simulink model "bldc0"  (R2022b)
settings: Solver=ode1  StartTime=0.0  StopTime=0.2  FixedStep=ctrlConst.TsSwitch  MaxStep=1e-6  RelTol=1e-3  EnableMultiTasking=on
values from neighbouring files (symbols this model uses):
  f32_P_AngleCompCur = 5461.0    [bldc.sldd]
  f32_P_AngleCompVol = 1.5    [bldc.sldd]
  f32_P_CurMax_A = 43.0    [bldc.sldd]
  f32_P_DeadPrd = 80.0    [bldc.sldd]
  f32_P_FwcCurMax_A = 54.2    [bldc.sldd]
  f32_P_fwcKi = 0.3    [bldc.sldd]
  f32_P_fwcKp = 11.0    [bldc.sldd]
  f32_P_IdInIF_A = -5.0    [bldc.sldd]
  f32_P_IdKi = 0.00010825    [bldc.sldd]
  f32_P_IdKp = 0.02    [bldc.sldd]
  f32_P_IdqFilter = 1250.0    [bldc.sldd]
  f32_P_IqKi = 0.00010825    [bldc.sldd]
  f32_P_IqKp = 0.02    [bldc.sldd]
  f32_P_MaxTrq_Nm = 1500.0    [bldc.sldd]
  f32_P_MinTrq_Nm = -1500.0    [bldc.sldd]
  f32_P_Modulation = 0.95    [bldc.sldd]
  f32_P_MotorPhi = 0.0026    [bldc.sldd]
  f32_P_PWMFreq = 10000.0    [bldc.sldd]
  f32_P_SpdNegKi = 10.0    [bldc.sldd]
  f32_P_SpdNegKp = 100.0    [bldc.sldd]
  f32_P_SpdNeglimit_rpm = -6000.0    [bldc.sldd]
  f32_P_SpdPosKi = 10.0    [bldc.sldd]
  f32_P_SpdPosKp = 100.0    [bldc.sldd]
  f32_P_SpdPoslimit_rpm = 6000.0    [bldc.sldd]
  f32_P_SpeedKi = 2.5E-6    [bldc.sldd]
  f32_P_SpeedKp = 0.02    [bldc.sldd]
  f32_P_SpeedPiMax = 1.5    [bldc.sldd]
  f32_P_SpeedPiMin = -1.5    [bldc.sldd]
  f32_P_Uqmax = 0.955    [bldc.sldd]
  u16_P_MotorPair = 4.0    [bldc.sldd]
undefined symbols (not defined in the file or in its folder): ECM
libraries: simulink x6, spsabctodq0Lib x1
(part 1 of 2)
settings Model: Creator=M00039784  LastModifiedBy=M00039784
settings SolverCC: AlgebraicLoopSolver=TrustRegion  InsertRTBMode=Never (minimum delay)
settings DataIOCC: LimitDataPoints=on  SaveFormat=Array  SaveOutput=off  SaveTime=off
settings OptimizationCC: DefaultParameterBehavior=Inlined  UseDivisionForNetSlopeComputation=on  UseFloatMulNetSlope=on  DefaultUnderspecifiedDataType=single  InlineInvariantSignals=on  PassReuseOutputArgsAs=Individual arguments  ExpressionDepthLimit=2147483647  ZeroExternalMemoryAtStartup=off  ZeroInternalMemoryAtStartup=off  NoFixptDivByZeroProtection=on  EfficientFloat2IntCast=on  LifeSpan=1  EfficientTunableParamExpr=on
settings DebuggingCC: ReadBeforeWriteMsg=DisableAll  WriteAfterWriteMsg=DisableAll  WriteAfterReadMsg=DisableAll  AlgebraicLoopMsg=none  MultiTaskDSMMsg=none  SingleTaskRateTransMsg=error  IntegerOverflowMsg=none  ParameterPrecisionLossMsg=none  FcnCallInpInsideContextMsg=warning  BusObjectLabelMismatch=none  AssertControl=DisableAll  AllowSymbolicDim=off  StateNameClashWarn=warning  SFUnexpectedBacktrackingDiag=warning  SFNoUnconditionalDefaultTransitionDiag=warning  SFExecutionAtInitializationDiag=none  SFMachineParentedDataDiag=warning  IntegerSaturationMsg=none  UnitsInconsistencyMsg=none  ArithmeticOperatorsInVariantConditions=warning
settings HardwareCC: ProdBitPerPointer=32  ProdBitPerSizeT=32  ProdBitPerPtrDiffT=32  ProdLargestAtomicFloat=None  ProdWordSize=32  ProdHWDeviceType=Infineon->TriCore
settings ModelReferenceCC: UpdateModelReferenceTargets=IfOutOfDate  EnableRefExpFcnMdlSchedulingChecks=on  ModelReferenceNumInstancesAllowed=Single  PropagateSignalLabelsOutOfModel=off
settings SFSimCC: SFSimEcho=off  SimUseLocalCustomCode=off  SimGenImportedTypeDefs=on  MATLABDynamicMemAlloc=off  CustomCodeUndefinedFunction=UseInterfaceOnly
settings RTWCC: Description=Embedded Coder  SystemTargetFile=ert.tlc  GenCodeOnly=on  GenerateMakefile=off  TemplateMakefile=ec_target.tmf  RTWVerbose=off  RTWUseLocalCustomCode=off  PortableWordSizes=on  CodeExecutionProfiling=on  CodeProfilingSaveOptions=AllData  CodeProfilingInstrumentation=detailed
settings CodeAppCC: ForceParamTrailComments=on  IgnoreCustomStorageClasses=off  IgnoreTestpoints=on  MaxIdLength=64  SimulinkDataObjDesc=on  MATLABFcnDesc=on  CustomSymbolStrGlobalVar=pmsmfoc_rt$N$M  CustomSymbolStrType=pmsmfoc_$N$M  CustomSymbolStrFcn=$N$M$F  CustomSymbolStrFcnArg=$I$N$M  CustomSymbolStrMacro=$N$M  InsertBlockDesc=on  StateflowObjectComments=on  MATLABSourceComments=on  InternalIdentifier=Classic
settings ERTTargetCC: UtilityFuncGeneration=Shared location  MultiwordLength=2048  CombineSignalStateStructs=on  SupportAbsoluteTime=off  SupportNonFinite=off  SupportComplex=off  SupportNonInlinedSFcns=on  RemoveResetFunc=off  ParenthesesLevel=Maximum  GenerateASAP2=on  InlinedParameterPlacement=NonHierarchical  ERTCustomFileTemplate=example_file_process.tlc  EnableDataOwnership=on  ConvertIfToSwitch=off  SuppressUnreachableDefaultCases=off  MemSecPackage=Simulink  MemSecDataConstants=MemConst  MemSecDataParameters=MemConstVolatile
settings ConfigComp: CovMetricSettings=dcmtrzow  CovHTMLOptions=-aTS=1 -bRG=1 -bTC=1 -hTR=0 -nFC=0 -scm=1 -bcm=1 -xEv=0  CovSaveCumulativeToWorkspaceVar=on  CovSaveSingleToWorkspaceVar=on  CovExternalEMLEnable=off  CovSFcnEnable=off
settings SimscapeCC: SimscapeNormalizeSystem=off

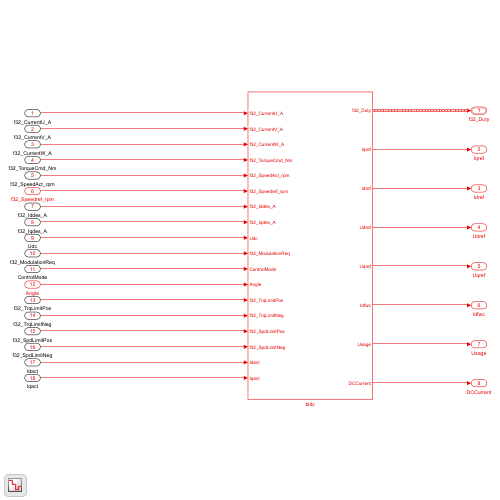
[thumbnail: Simulink's stored preview of the top-level diagram]
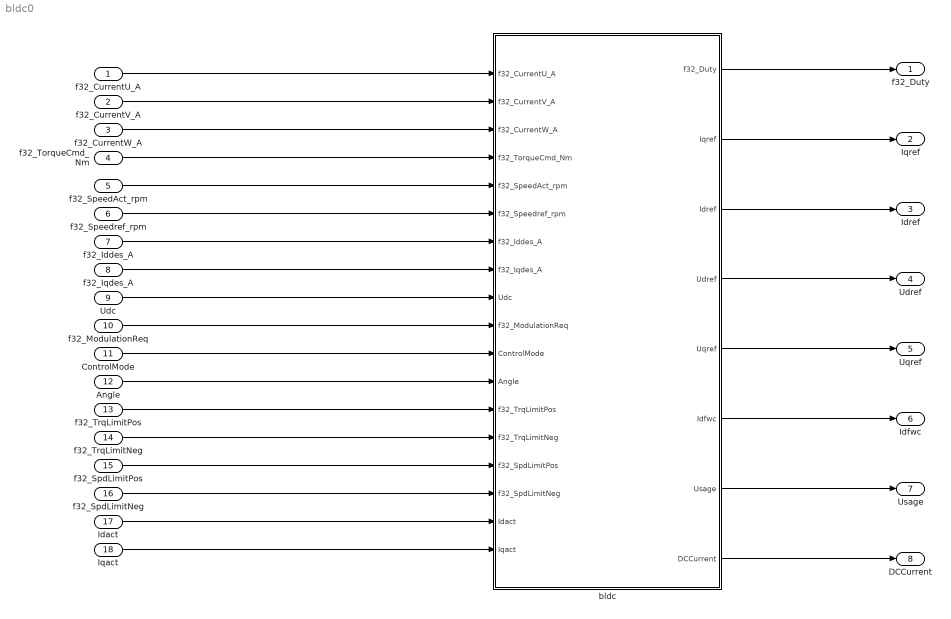
== system bldc0 ==
  f32_CurrentU_A : Inport  OutDataTypeStr=single  PortDimensions=1  SampleTime=0.0001
  f32_CurrentV_A : Inport  Port=2  OutDataTypeStr=single  PortDimensions=1  SampleTime=0.0001
  f32_CurrentW_A : Inport  Port=3  OutDataTypeStr=single  PortDimensions=1  SampleTime=0.0001
  f32_TorqueCmd_Nm : Inport  Port=4  OutDataTypeStr=single  PortDimensions=1
  f32_SpeedAct_rpm : Inport  Port=5  OutDataTypeStr=single  PortDimensions=1  SampleTime=0.0001
  f32_Speedref_rpm : Inport  Port=6  OutDataTypeStr=single  PortDimensions=1
  f32_Iddes_A : Inport  Port=7
  f32_Iqdes_A : Inport  Port=8
  "Udc " : Inport  Port=9  OutDataTypeStr=single  PortDimensions=1
  f32_ModulationReq : Inport  Port=10  OutDataTypeStr=single  PortDimensions=1
  ControlMode : Inport  Port=11  OutDataTypeStr=Enum: ECM  PortDimensions=1  SampleTime=0.0001
  Angle : Inport  Port=12  OutDataTypeStr=uint16  PortDimensions=1  SampleTime=0.0001
  f32_TrqLimitPos : Inport  Port=13
  f32_TrqLimitNeg : Inport  Port=14
  f32_SpdLimitPos : Inport  Port=15
  f32_SpdLimitNeg : Inport  Port=16
  Idact : Inport  Port=17
  Iqact : Inport  Port=18
  bldc : Subsystem
  f32_Duty : Outport  OutDataTypeStr=Bus: Duty
  Iqref : Outport  Port=2
  Idref : Outport  Port=3
  Udref : Outport  Port=4
  Uqref : Outport  Port=5
  Idfwc : Outport  Port=6
  Usage : Outport  Port=7
  DCCurrent : Outport  Port=8
  wires:
  f32_CurrentU_A/1 -> bldc/1(f32_CurrentU_A)
  f32_CurrentV_A/1 -> bldc/2(f32_CurrentV_A)
  f32_CurrentW_A/1 -> bldc/3(f32_CurrentW_A)
  f32_TorqueCmd_Nm/1 -> bldc/4(f32_TorqueCmd_Nm)
  f32_SpeedAct_rpm/1 -> bldc/5(f32_SpeedAct_rpm)
  f32_Speedref_rpm/1 -> bldc/6(f32_Speedref_rpm)
  "Udc "/1 -> bldc/9("Udc ")
  f32_ModulationReq/1 -> bldc/10(f32_ModulationReq)
  ControlMode/1 -> bldc/11(ControlMode)
  Angle/1 -> bldc/12(Angle)
  f32_TrqLimitPos/1 -> bldc/13(f32_TrqLimitPos)
  f32_TrqLimitNeg/1 -> bldc/14(f32_TrqLimitNeg)
  f32_SpdLimitPos/1 -> bldc/15(f32_SpdLimitPos)
  f32_SpdLimitNeg/1 -> bldc/16(f32_SpdLimitNeg)
  bldc/1(f32_Duty) -> f32_Duty/1
  bldc/2(Iqref) -> Iqref/1
  bldc/3(Idref) -> Idref/1
  bldc/4(Udref) -> Udref/1
  bldc/5(Uqref) -> Uqref/1
  bldc/6(Idfwc) -> Idfwc/1
  bldc/7(Usage) -> Usage/1
  bldc/8(DCCurrent) -> DCCurrent/1
  f32_Iddes_A/1 -> bldc/7(f32_Iddes_A)
  f32_Iqdes_A/1 -> bldc/8(f32_Iqdes_A)
  Idact/1 -> bldc/17(Idact)
  Iqact/1 -> bldc/18(Iqact)

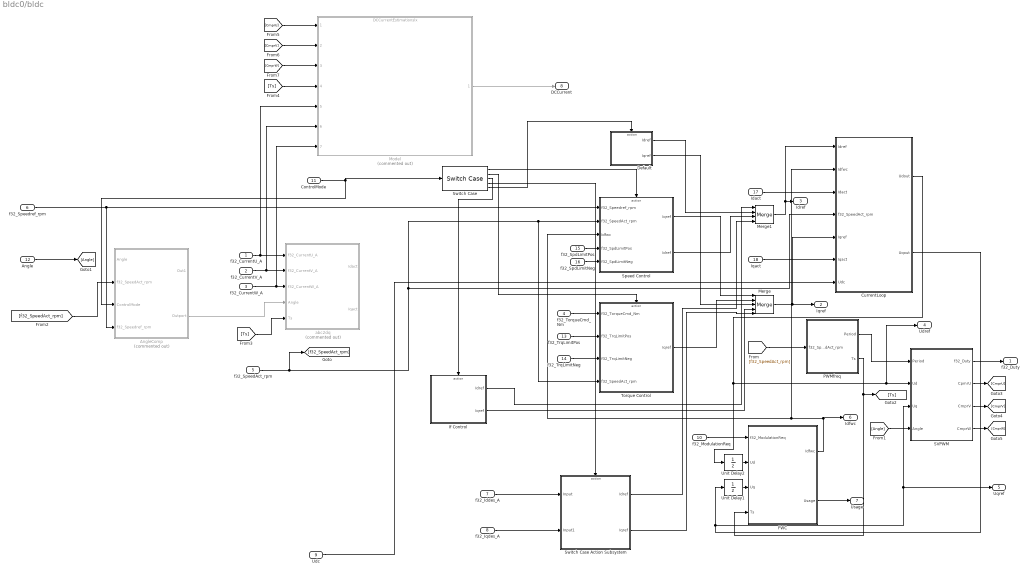
== system bldc0/bldc ==
  f32_CurrentU_A : Inport  OutDataTypeStr=single  PortDimensions=1  SampleTime=0.0001
  f32_CurrentV_A : Inport  Port=2  OutDataTypeStr=single  PortDimensions=1  SampleTime=0.0001
  f32_CurrentW_A : Inport  Port=3  OutDataTypeStr=single  PortDimensions=1  SampleTime=0.0001
  f32_TorqueCmd_Nm : Inport  Port=4  OutDataTypeStr=single  PortDimensions=1
  f32_SpeedAct_rpm : Inport  Port=5  OutDataTypeStr=single  PortDimensions=1  SampleTime=0.0001
  f32_Speedref_rpm : Inport  Port=6  OutDataTypeStr=single  PortDimensions=1  SampleTime=0.0001
  f32_Iddes_A : Inport  Port=7
  f32_Iqdes_A : Inport  Port=8
  "Udc " : Inport  Port=9  OutDataTypeStr=single  PortDimensions=1
  f32_ModulationReq : Inport  Port=10  OutDataTypeStr=single  PortDimensions=1
  ControlMode : Inport  Port=11  OutDataTypeStr=Enum: ECM  PortDimensions=1  SampleTime=0.0001
  Angle : Inport  Port=12  OutDataTypeStr=uint16  PortDimensions=1  SampleTime=0.0001
  f32_TrqLimitPos : Inport  Port=13
  f32_TrqLimitNeg : Inport  Port=14
  f32_SpdLimitPos : Inport  Port=15
  f32_SpdLimitNeg : Inport  Port=16
  Idact : Inport  Port=17
  Iqact : Inport  Port=18
  AngleComp : Subsystem  Commented=on  TreatAsAtomicUnit=on
  CurrentLoop : Subsystem
  Default : Subsystem  TreatAsAtomicUnit=on
  FWC : Subsystem
  If Control : Subsystem  TreatAsAtomicUnit=on
  Merge : Merge  Inputs=5  InitialOutput=0
  Merge1 : Merge  Inputs=4  InitialOutput=0
  Model : ModelReference  Commented=on  ModelNameDialog=DCCurrentEstimationslx.slx  SimulationMode=Normal  ModelReferenceVersion=1.34
  PWMfreq : Subsystem
  SVPWM : Subsystem
  Speed Control : Subsystem
  Switch Case : SwitchCase  CaseConditions={ECM.nCtrl,ECM.TrqCtrl,ECM.IFCtrl,ECM.IsCtrl}
  Switch Case Action Subsystem : Subsystem  TreatAsAtomicUnit=on
  Torque Control : Subsystem
  Unit Delay1 : UnitDelay  SampleTime=-1  HasFrameUpgradeWarning=on
  Unit Delay2 : UnitDelay  SampleTime=-1  HasFrameUpgradeWarning=on
  abc2dq : Subsystem  Commented=on
  f32_Duty : Outport  OutDataTypeStr=Bus: Duty
  Iqref : Outport  Port=2
  Idref : Outport  Port=3
  Udref : Outport  Port=4
  Uqref : Outport  Port=5
  Idfwc : Outport  Port=6
  Usage : Outport  Port=7
  DCCurrent : Outport  Port=8
  wires:
  SVPWM/1(f32_Duty) -> f32_Duty/1
  PWMfreq/1(Period) -> SVPWM/1(Period)
  f32_CurrentW_A/1 -> Model/7, abc2dq/3(f32_CurrentW_A)
  CurrentLoop/1("Udout ") -> Unit Delay2/1, Udref/1, SVPWM/2(Ud)
  [Angle] -> SVPWM/4(Angle)
  f32_CurrentU_A/1 -> Model/5, abc2dq/1(f32_CurrentU_A)
  f32_SpeedAct_rpm/1 -> CurrentLoop/4(f32_SpeedAct_rpm), Torque Control/4(f32_SpeedAct_rpm), Speed Control/2(f32_SpeedAct_rpm), [f32_SpeedAct_rpm]
  f32_TorqueCmd_Nm/1 -> Torque Control/1(f32_TorqueCmd_Nm)
  f32_SpdLimitPos/1 -> Speed Control/4(f32_SpdLimitPos)
  Switch Case/2 -> Torque Control/Action
  Merge/1 -> CurrentLoop/5(Iqref), Iqref/1
  FWC/1(Idfwc) -> Idfwc/1, CurrentLoop/2(Idfwc), Speed Control/3(Idfwc)
  f32_CurrentV_A/1 -> Model/6, abc2dq/2(f32_CurrentV_A)
  f32_SpdLimitNeg/1 -> Speed Control/5(f32_SpdLimitNeg)
  Speed Control/1("Iqref ") -> Merge/1
  Switch Case/3 -> If Control/Action
  f32_Speedref_rpm/1 -> AngleComp/4(f32_Speedref_rpm), Speed Control/1(f32_Speedref_rpm)
  If Control/1(Idref) -> Merge1/1
  FWC/2(Usage) -> Usage/1
  CurrentLoop/2(Uqout) -> Unit Delay1/1, Uqref/1, SVPWM/3(Uq)
  f32_TrqLimitPos/1 -> Torque Control/2(f32_TrqLimitPos)
  PWMfreq/2(Ts) -> FWC/4(Ts), [Ts]
  Default/1("Idref ") -> Merge1/2
  AngleComp/2(Outport) -> abc2dq/4(Angle)
  Unit Delay1/1 -> FWC/3(Uq)
  [f32_SpeedAct_rpm] -> AngleComp/2(f32_SpeedAct_rpm)
  Merge1/1 -> CurrentLoop/1(Idref), Idref/1
  Switch Case/5 -> Default/Action
  [f32_SpeedAct_rpm] -> PWMfreq/1(f32_SpeedAct_rpm)
  f32_TrqLimitNeg/1 -> Torque Control/3(f32_TrqLimitNeg)
  Default/2(Iqref) -> Merge/3
  ControlMode/1 -> AngleComp/3(ControlMode), Switch Case/1
  Switch Case/1 -> Speed Control/Action
  Angle/1 -> [Angle]
  If Control/2(Iqref) -> Merge/4
  Torque Control/1(Iqref) -> Merge/2
  Idact/1 -> CurrentLoop/3(Idact)
  "Udc "/1 -> CurrentLoop/7("Udc ")
  f32_ModulationReq/1 -> FWC/1(f32_ModulationReq)
  Speed Control/2(Idref) -> Merge1/3
  Iqact/1 -> CurrentLoop/6(Iqact)
  [Ts] -> abc2dq/5(Ts)
  Unit Delay2/1 -> FWC/2(Ud)
  [Ts] -> Model/4
  SVPWM/2(CpmrU) -> [CmprU]
  SVPWM/3(CmprV) -> [CmprV]
  SVPWM/4(CmprW) -> [CmprW]
  [CmprW] -> Model/3
  [CmprV] -> Model/2
  [CmprU] -> Model/1
  Model/1 -> DCCurrent/1
  f32_Iddes_A/1 -> Switch Case Action Subsystem/1(Input)
  f32_Iqdes_A/1 -> Switch Case Action Subsystem/2(Input1)
  Switch Case Action Subsystem/1("Idref ") -> Merge1/4
  Switch Case Action Subsystem/2(Iqref) -> Merge/5
  Switch Case/4 -> Switch Case Action Subsystem/Action

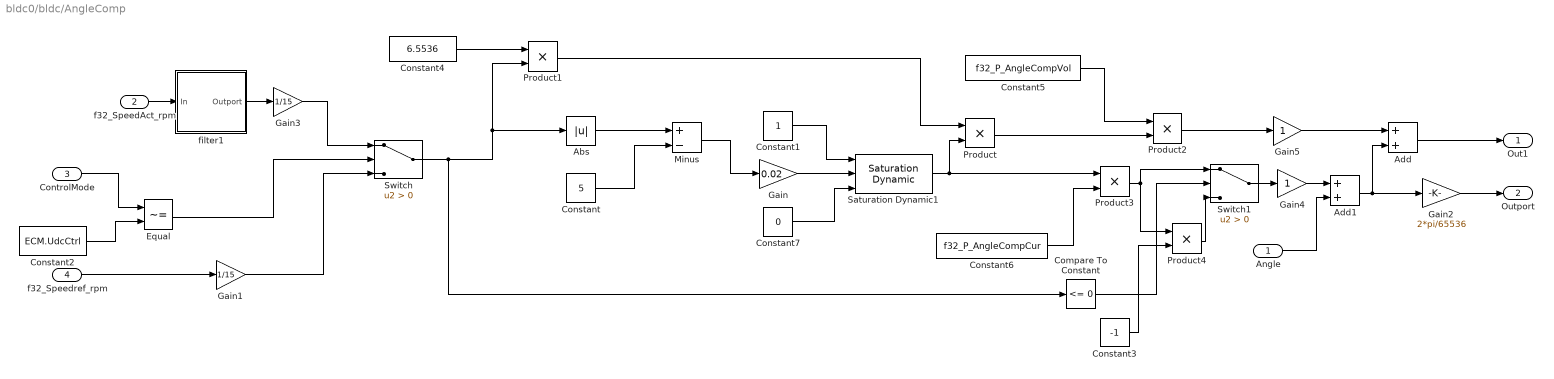
== system bldc0/bldc/AngleComp ==
  Angle : Inport
  f32_SpeedAct_rpm : Inport  Port=2
  ControlMode : Inport  Port=3
  f32_Speedref_rpm : Inport  Port=4
  Abs : Abs  SaturateOnIntegerOverflow=off
  Add : Sum  OutDataTypeStr=uint16
  Add1 : Sum  AccumDataTypeStr=uint16
  Compare To Constant : simulink/Logic and Bit Operations/Compare To Constant  relop=<=  const=0  OutDataTypeStr=boolean
  Constant : Constant  Value=5  OutDataTypeStr=single
  Constant1 : Constant  OutDataTypeStr=single
  Constant2 : Constant  Value=ECM.UdcCtrl  OutDataTypeStr=Enum: ECM
  Constant3 : Constant  Value=-1
  Constant4 : Constant  Value=6.5536  OutDataTypeStr=single
  Constant5 : Constant  Value=f32_P_AngleCompVol
  Constant6 : Constant  Value=f32_P_AngleCompCur
  Constant7 : Constant  Value=0  OutDataTypeStr=single
  Equal : RelationalOperator  Operator=~=  OutDataTypeStr=boolean  RndMeth=Simplest  InputSameDT=off
  Gain : Gain  Gain=0.02
  Gain1 : Gain  Gain=1/15  ParamDataTypeStr=single
  Gain2 : Gain  Gain=2*pi/65536  OutDataTypeStr=single
  Gain3 : Gain  Gain=1/15  ParamDataTypeStr=single
  Gain4 : Gain  OutDataTypeStr=uint16
  Gain5 : Gain  OutDataTypeStr=uint16
  Minus : Sum  Inputs=+-
  Product{,1,3..4} (4 alike) : Product  OutDataTypeStr=single
  Product2 : Product  OutDataTypeStr=int16
  Saturation Dynamic1 : simulink/Discontinuities/Saturation Dynamic  OutMin=[]  OutMax=[]  OutDataTypeStr=Inherit: Same as second input  OutDataType=fixdt(1, 16)  OutScaling=2^-10  DoSatur=off
  Switch : Switch  Criteria=u2 > Threshold  OutDataTypeStr=single  SaturateOnIntegerOverflow=off  InputSameDT=off
  Switch1 : Switch  Criteria=u2 > Threshold  OutDataTypeStr=int16  SaturateOnIntegerOverflow=off  InputSameDT=off
  filter1 : Subsystem
  Out1 : Outport
  Outport : Outport  Port=2  OutDataTypeStr=single
  wires:
  f32_SpeedAct_rpm/1 -> filter1/1(In)
  Abs/1 -> Minus/1
  Constant/1 -> Minus/2
  Product1/1 -> Product/1
  Constant4/1 -> Product1/1
  Constant5/1 -> Product2/1
  Product/1 -> Product2/2
  Constant6/1 -> Product3/2
  Product2/1 -> Gain5/1
  Gain4/1 -> Add1/1
  Angle/1 -> Add1/2
  Add1/1 -> Gain2/1, Add/2
  Add/1 -> Out1/1
  Gain2/1 -> Outport/1
  Constant7/1 -> Saturation Dynamic1/3
  Constant1/1 -> Saturation Dynamic1/1
  Minus/1 -> Gain/1
  Gain/1 -> Saturation Dynamic1/2
  Switch/1 -> Compare To Constant/1, Abs/1, Product1/2
  filter1/1(Outport) -> Gain3/1
  ControlMode/1 -> Equal/1
  Constant2/1 -> Equal/2
  Equal/1 -> Switch/2
  f32_Speedref_rpm/1 -> Gain1/1
  Saturation Dynamic1/1 -> Product3/1, Product/2
  Compare To Constant/1 -> Switch1/2
  Product3/1 -> Switch1/1, Product4/1
  Product4/1 -> Switch1/3
  Constant3/1 -> Product4/2
  Gain1/1 -> Switch/3
  Gain3/1 -> Switch/1
  Switch1/1 -> Gain4/1
  Gain5/1 -> Add/1

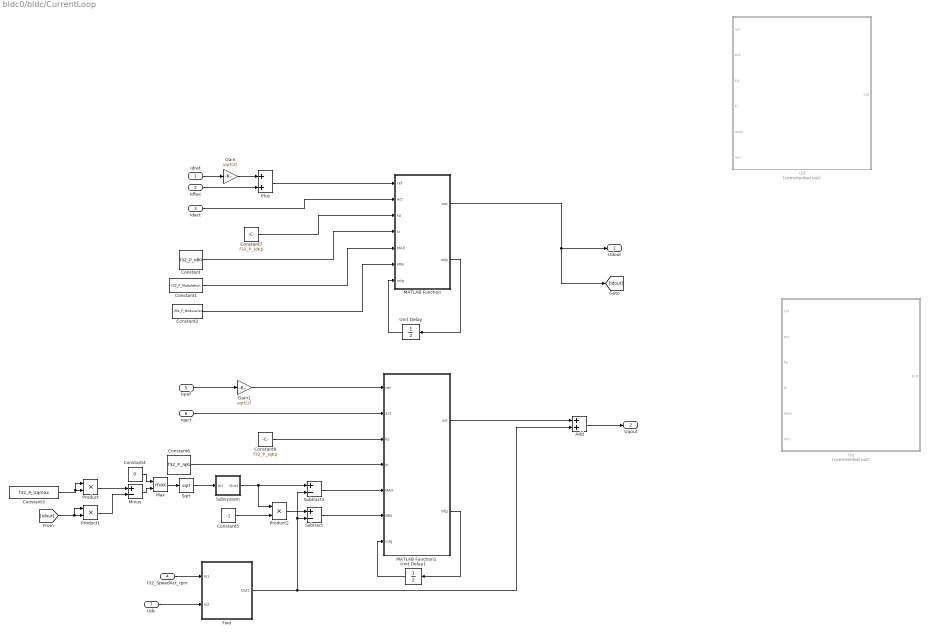
== system bldc0/bldc/CurrentLoop ==
  Idref : Inport
  Idfwc : Inport  Port=2
  Idact : Inport  Port=3
  f32_SpeedAct_rpm : Inport  Port=4
  Iqref : Inport  Port=5
  Iqact : Inport  Port=6
  "Udc " : Inport  Port=7
  Add : Sum
  Constant : Constant  Value=f32_P_IdKi
  Constant1 : Constant  Value=f32_P_Modulation
  Constant2 : Constant  Value=-f32_P_Modulation
  Constant3 : Constant  Value=f32_P_Uqmax
  Constant4 : Constant  Value=0  OutDataTypeStr=single
  Constant5 : Constant  Value=-1  OutDataTypeStr=single
  Constant6 : Constant  Value=f32_P_IqKi
  Constant7 : Constant  Value=f32_P_IdKp
  Constant8 : Constant  Value=f32_P_IqKp
  Fwd : Subsystem
  Gain : Gain  Gain=sqrt(2)
  Gain1 : Gain  Gain=sqrt(2)
  MATLAB Function : MATLAB Function  TreatAsAtomicUnit=on
  MATLAB Function1 : MATLAB Function  TreatAsAtomicUnit=on
  Max : MinMax  Function=max  Inputs=2
  Minus : Sum  Inputs=+-
  Plus : Sum
  Product : Product
  Product1 : Product
  Product2 : Product
  Sqrt : Sqrt
  Subsystem : Subsystem
  Subtract : Sum  Inputs=+-
  Subtract1 : Sum  Inputs=+-
  Ud : Stateflow chart  Commented=on  TreatAsAtomicUnit=on
  Unit Delay : UnitDelay  SampleTime=-1  HasFrameUpgradeWarning=on
  Unit Delay1 : UnitDelay  SampleTime=-1  HasFrameUpgradeWarning=on
  Uq : Stateflow chart  Commented=on  TreatAsAtomicUnit=on
  "Udout " : Outport
  Uqout : Outport  Port=2  VectorParamsAs1DForOutWhenUnconnected=off
  wires:
  MATLAB Function1/1(out) -> Add/1
  Add/1 -> Uqout/1
  Subtract1/1 -> MATLAB Function1/5(MAX)
  Fwd/1(Out1) -> Subtract/2, Subtract1/2, Add/2
  Subtract/1 -> MATLAB Function1/6(MIN)
  Product2/1 -> Subtract/1
  "Udc "/1 -> Fwd/2(In2)
  f32_SpeedAct_rpm/1 -> Fwd/1(In1)
  Constant6/1 -> MATLAB Function1/4(ki)
  Constant8/1 -> MATLAB Function1/3(kp)
  Constant5/1 -> Product2/2
  Subsystem/1(Out1) -> Subtract1/1, Product2/1
  Sqrt/1 -> Subsystem/1(In1)
  Constant4/1 -> Max/1
  Max/1 -> Sqrt/1
  Minus/1 -> Max/2
  Product1/1 -> Minus/2
  [Idout] -> Product1/2, Product1/1
  Product/1 -> Minus/1
  Constant3/1 -> Product/2, Product/1
  Iqact/1 -> MATLAB Function1/2(act)
  Iqref/1 -> Gain1/1
  Idref/1 -> Gain/1
  MATLAB Function/1(out) -> [Idout], "Udout "/1
  Constant2/1 -> MATLAB Function/6(MIN)
  Constant1/1 -> MATLAB Function/5(MAX)
  Constant/1 -> MATLAB Function/4(ki)
  Constant7/1 -> MATLAB Function/3(kp)
  Idact/1 -> MATLAB Function/2(act)
  Plus/1 -> MATLAB Function/1(ref)
  Idfwc/1 -> Plus/2
  Gain/1 -> Plus/1
  Gain1/1 -> MATLAB Function1/1(ref)
  MATLAB Function/2(intg) -> Unit Delay/1
  Unit Delay/1 -> MATLAB Function/7("intg ")
  Unit Delay1/1 -> MATLAB Function1/7("intg ")
  MATLAB Function1/2(intg) -> Unit Delay1/1

== system bldc0/bldc/Default ==
  Action Port : ActionPort  InitializeStates=reset  ActionPortLabel=default:
  Constant : Constant  Value=0  OutDataTypeStr=single
  Constant1 : Constant  Value=0  OutDataTypeStr=single
  "Idref " : Outport  VectorParamsAs1DForOutWhenUnconnected=off
  Iqref : Outport  Port=2  VectorParamsAs1DForOutWhenUnconnected=off
  wires:
  Constant1/1 -> Iqref/1
  Constant/1 -> "Idref "/1

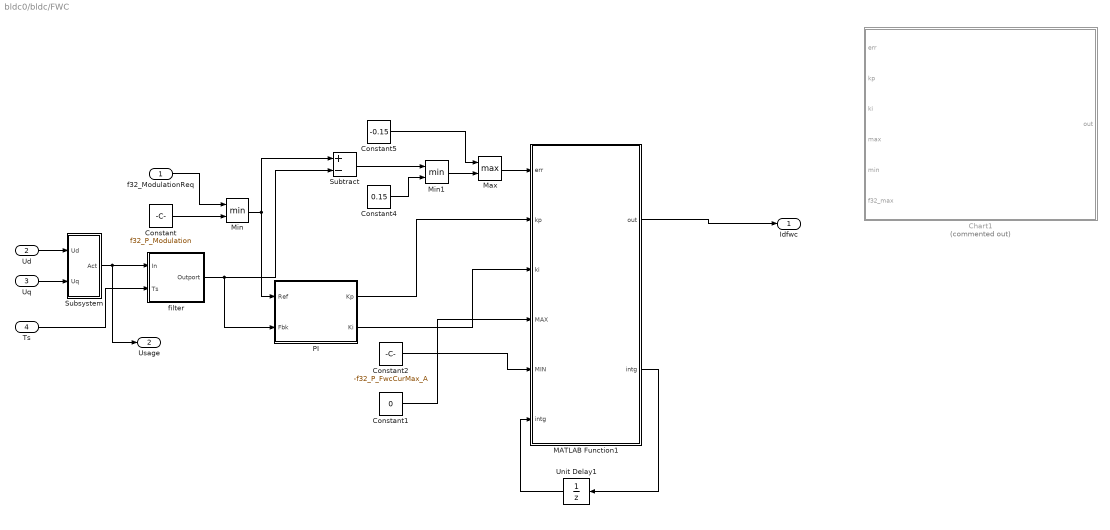
== system bldc0/bldc/FWC ==
  f32_ModulationReq : Inport
  Ud : Inport  Port=2
  Uq : Inport  Port=3
  Ts : Inport  Port=4
  Chart1 : Stateflow chart  Commented=on  TreatAsAtomicUnit=on
  Constant : Constant  Value=f32_P_Modulation  OutDataTypeStr=single
  Constant1 : Constant  Value=0  OutDataTypeStr=single
  Constant2 : Constant  Value=-f32_P_FwcCurMax_A  OutDataTypeStr=single
  Constant4 : Constant  Value=0.15  OutDataTypeStr=single
  Constant5 : Constant  Value=-0.15  OutDataTypeStr=single
  MATLAB Function1 : MATLAB Function  TreatAsAtomicUnit=on
  Max : MinMax  Function=max  Inputs=2
  Min : MinMax  Inputs=2
  Min1 : MinMax  Inputs=2
  PI : Subsystem
  Subsystem : Subsystem
  Subtract : Sum  Inputs=+-
  Unit Delay1 : UnitDelay  SampleTime=-1  HasFrameUpgradeWarning=on
  filter : Subsystem
  Idfwc : Outport  VectorParamsAs1DForOutWhenUnconnected=off
  Usage : Outport  Port=2
  wires:
  Max/1 -> MATLAB Function1/1(err)
  Constant5/1 -> Max/1
  Min1/1 -> Max/2
  Constant4/1 -> Min1/2
  Subtract/1 -> Min1/1
  Constant1/1 -> MATLAB Function1/4(MAX)
  PI/2(Ki) -> MATLAB Function1/3(ki)
  PI/1(Kp) -> MATLAB Function1/2(kp)
  Constant2/1 -> MATLAB Function1/5(MIN)
  Subsystem/1(Act) -> Usage/1, filter/1(In)
  Uq/1 -> Subsystem/2(Uq)
  Ud/1 -> Subsystem/1(Ud)
  Min/1 -> Subtract/1, PI/1(Ref)
  Constant/1 -> Min/2
  f32_ModulationReq/1 -> Min/1
  MATLAB Function1/1(out) -> Idfwc/1
  filter/1(Outport) -> Subtract/2, PI/2(Fbk)
  MATLAB Function1/2(intg) -> Unit Delay1/1
  Unit Delay1/1 -> MATLAB Function1/6("intg ")
  Ts/1 -> filter/2(Ts)

== system bldc0/bldc/If Control ==
  Action Port : ActionPort  InitializeStates=reset  ActionPortLabel=case [ IFCtrl ]:
  Constant : Constant  Value=f32_P_IdInIF_A  OutDataTypeStr=single
  Constant1 : Constant  Value=0  OutDataTypeStr=single
  Idref : Outport  InitialOutput=0  VectorParamsAs1DForOutWhenUnconnected=off
  Iqref : Outport  Port=2  InitialOutput=0
  wires:
  Constant/1 -> Idref/1
  Constant1/1 -> Iqref/1

== system bldc0/bldc/PWMfreq ==
  f32_SpeedAct_rpm : Inport
  1-D Lookup Table : Lookup_n-D  Commented=on  NumberOfTableDimensions=1  BreakpointsForDimension1=[0 400 800]  Table=[5000;5000;5000]  InternalRulePriority=Speed  OutDataTypeStr=uint32  RndMeth=Simplest
  Constant : Constant  Value=f32_P_PWMFreq  OutDataTypeStr=single
  Constant1 : Constant  OutDataTypeStr=single
  Divide : Product  Inputs=*/
  Gain : Gain  Gain=100000000  OutDataTypeStr=uint32
  Period : Outport  OutDataTypeStr=uint32  VectorParamsAs1DForOutWhenUnconnected=off
  Ts : Outport  Port=2  OutDataTypeStr=single
  wires:
  Constant/1 -> Divide/2
  f32_SpeedAct_rpm/1 -> 1-D Lookup Table/1
  Divide/1 -> Gain/1, Ts/1
  Constant1/1 -> Divide/1
  Gain/1 -> Period/1

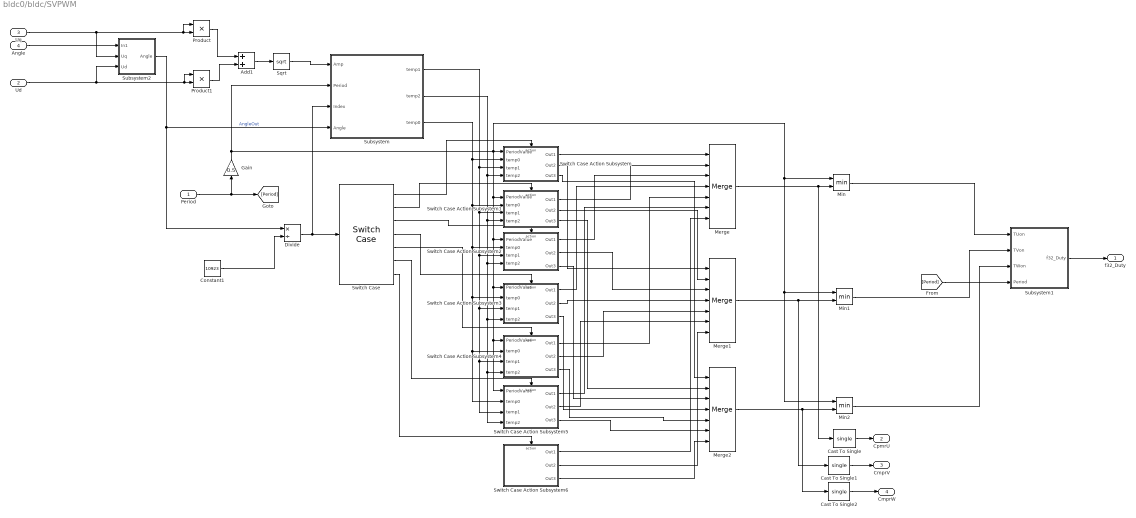
== system bldc0/bldc/SVPWM ==
  Period : Inport
  Ud : Inport  Port=2
  Uq : Inport  Port=3
  Angle : Inport  Port=4  OutDataTypeStr=uint16
  Add1 : Sum  OutDataTypeStr=single
  Cast To Single : DataTypeConversion  OutDataTypeStr=single  SaturateOnIntegerOverflow=off  RndMeth=Floor
  Cast To Single1 : DataTypeConversion  OutDataTypeStr=single  SaturateOnIntegerOverflow=off  RndMeth=Floor
  Cast To Single2 : DataTypeConversion  OutDataTypeStr=single  SaturateOnIntegerOverflow=off  RndMeth=Floor
  Constant1 : Constant  Value=10923  OutDataTypeStr=single
  Divide : Product  Inputs=*/  OutDataTypeStr=uint16
  Gain : Gain  Gain=0.5
  Merge : Merge  Inputs=7
  Merge1 : Merge  Inputs=7
  Merge2 : Merge  Inputs=7
  Min : MinMax  Inputs=2
  Min1 : MinMax  Inputs=2
  Min2 : MinMax  Inputs=2
  Product : Product  OutDataTypeStr=single
  Product1 : Product  OutDataTypeStr=single
  Sqrt : Sqrt  OutDataTypeStr=single
  Subsystem : Subsystem
  Subsystem1 : Subsystem
  Subsystem2 : Subsystem
  Switch Case : SwitchCase  CaseConditions={0,1,2,3,4,5}
  Switch Case Action Subsystem : Subsystem  TreatAsAtomicUnit=on
  Switch Case Action Subsystem1 : Subsystem  TreatAsAtomicUnit=on
  Switch Case Action Subsystem2 : Subsystem  TreatAsAtomicUnit=on
  Switch Case Action Subsystem3 : Subsystem  TreatAsAtomicUnit=on
  Switch Case Action Subsystem4 : Subsystem  TreatAsAtomicUnit=on
  Switch Case Action Subsystem5 : Subsystem  TreatAsAtomicUnit=on
  Switch Case Action Subsystem6 : Subsystem  TreatAsAtomicUnit=on
  f32_Duty : Outport  OutDataTypeStr=Bus: Duty
  CpmrU : Outport  Port=2
  CmprV : Outport  Port=3
  CmprW : Outport  Port=4
  wires:
  Add1/1 -> Sqrt/1
  Product1/1 -> Add1/2
  Product/1 -> Add1/1
  Min2/1 -> Subsystem1/3(TWon)
  Min1/1 -> Subsystem1/2(TVon)
  Min/1 -> Subsystem1/1(TUon)
  Merge2/1 -> Cast To Single2/1, Min2/2
  Merge1/1 -> Cast To Single1/1, Min1/2
  Merge/1 -> Cast To Single/1, Min/2
  Subsystem/2(temp2) -> Switch Case Action Subsystem/4(temp2), Switch Case Action Subsystem1/4(temp2), Switch Case Action Subsystem2/4(temp2), Switch Case Action Subsystem4/4(temp2), Switch Case Action Subsystem5/4(temp2), Switch Case Action Subsystem3/4(temp2)
  Subsystem/1(temp1) -> Switch Case Action Subsystem/3(temp1), Switch Case Action Subsystem1/3(temp1), Switch Case Action Subsystem2/3(temp1), Switch Case Action Subsystem3/3(temp1), Switch Case Action Subsystem4/3(temp1), Switch Case Action Subsystem5/3(temp1)
  Subsystem/3(temp0) -> Switch Case Action Subsystem/2(temp0), Switch Case Action Subsystem1/2(temp0), Switch Case Action Subsystem2/2(temp0), Switch Case Action Subsystem3/2(temp0), Switch Case Action Subsystem4/2(temp0), Switch Case Action Subsystem5/2(temp0)
  Sqrt/1 -> Subsystem/1(Amp)
  Switch Case Action Subsystem/3(Out3) -> Merge2/1
  Switch Case Action Subsystem1/3(Out3) -> Merge2/2
  Switch Case Action Subsystem2/3(Out3) -> Merge2/3
  Switch Case Action Subsystem3/3(Out3) -> Merge2/4
  Switch Case Action Subsystem4/3(Out3) -> Merge2/5
  Switch Case Action Subsystem5/3(Out3) -> Merge2/6
  Switch Case Action Subsystem6/3(Out3) -> Merge2/7
  Switch Case Action Subsystem6/2(Out2) -> Merge1/7
  Switch Case Action Subsystem5/2(Out2) -> Merge1/6
  Switch Case Action Subsystem4/2(Out2) -> Merge1/5
  Switch Case Action Subsystem3/2(Out2) -> Merge1/4
  Switch Case Action Subsystem2/2(Out2) -> Merge1/3
  Switch Case Action Subsystem1/2(Out2) -> Merge1/2
  Switch Case Action Subsystem/2(Out2) -> Merge1/1
  Switch Case Action Subsystem6/1(Out1) -> Merge/7
  Switch Case Action Subsystem5/1(Out1) -> Merge/6
  Switch Case Action Subsystem4/1(Out1) -> Merge/5
  Switch Case Action Subsystem3/1(Out1) -> Merge/4
  Switch Case Action Subsystem2/1(Out1) -> Merge/3
  Switch Case Action Subsystem1/1(Out1) -> Merge/2
  Switch Case Action Subsystem/1(Out1) -> Merge/1
  Switch Case/7 -> Switch Case Action Subsystem6/Action
  Switch Case/6 -> Switch Case Action Subsystem5/Action
  Switch Case/5 -> Switch Case Action Subsystem4/Action
  Switch Case/4 -> Switch Case Action Subsystem3/Action
  Switch Case/3 -> Switch Case Action Subsystem2/Action
  Switch Case/2 -> Switch Case Action Subsystem1/Action
  Switch Case/1 -> Switch Case Action Subsystem/Action
  Divide/1 -> Subsystem/3(Index), Switch Case/1
  Constant1/1 -> Divide/2
  [Period] -> Subsystem1/4(Period)
  Subsystem1/1(f32_Duty) -> f32_Duty/1
  Angle/1 -> Subsystem2/1(In1)
  Uq/1 -> Product/2, Product/1, Subsystem2/2(Uq)
  Ud/1 -> Product1/1, Product1/2, Subsystem2/3(Ud)
  Subsystem2/1(Angle) -> Divide/1, Subsystem/4(Angle)  "AngleOut"
  Period/1 -> [Period], Gain/1
  Gain/1 -> Switch Case Action Subsystem/1(PeriodValue), Switch Case Action Subsystem1/1(PeriodValue), Switch Case Action Subsystem2/1(PeriodValue), Switch Case Action Subsystem3/1(PeriodValue), Switch Case Action Subsystem4/1(PeriodValue), Switch Case Action Subsystem5/1(PeriodValue), Min/1, Min1/1, Min2/1, Subsystem/2(Period)
  Cast To Single/1 -> CpmrU/1
  Cast To Single1/1 -> CmprV/1
  Cast To Single2/1 -> CmprW/1

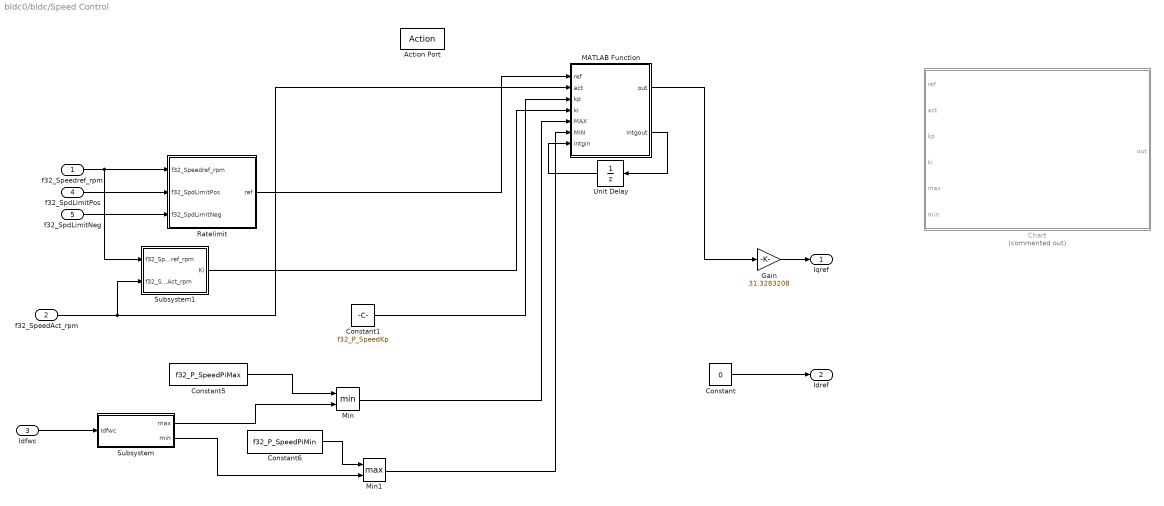
== system bldc0/bldc/Speed Control ==
  f32_Speedref_rpm : Inport
  f32_SpeedAct_rpm : Inport  Port=2
  Idfwc : Inport  Port=3
  f32_SpdLimitPos : Inport  Port=4
  f32_SpdLimitNeg : Inport  Port=5
  Action Port : ActionPort  InitializeStates=reset  ActionPortLabel=case [ nCtrl ]:
  Chart : Stateflow chart  Commented=on  TreatAsAtomicUnit=on
  Constant : Constant  Value=0  OutDataTypeStr=single
  Constant1 : Constant  Value=f32_P_SpeedKp
  Constant5 : Constant  Value=f32_P_SpeedPiMax
  Constant6 : Constant  Value=f32_P_SpeedPiMin
  Gain : Gain  Gain=31.3283208  OutDataTypeStr=single
  MATLAB Function : MATLAB Function  TreatAsAtomicUnit=on
  Min : MinMax  Inputs=2
  Min1 : MinMax  Function=max  Inputs=2
  Ratelimit : Subsystem
  Subsystem : Subsystem
  Subsystem1 : Subsystem
  Unit Delay : UnitDelay  SampleTime=-1  HasFrameUpgradeWarning=on
  "Iqref " : Outport  InitialOutput=0
  Idref : Outport  Port=2
  wires:
  f32_Speedref_rpm/1 -> Subsystem1/1(f32_Speedref_rpm), Ratelimit/1(f32_Speedref_rpm)
  Idfwc/1 -> Subsystem/1(Idfwc)
  Subsystem/2(min) -> Min1/2
  Constant6/1 -> Min1/1
  Subsystem/1(max) -> Min/2
  Constant5/1 -> Min/1
  MATLAB Function/1(out) -> Gain/1
  Min1/1 -> MATLAB Function/6(MIN)
  Min/1 -> MATLAB Function/5(MAX)
  Constant1/1 -> MATLAB Function/3(kp)
  f32_SpeedAct_rpm/1 -> MATLAB Function/2(act), Subsystem1/2(f32_SpeedAct_rpm)
  Ratelimit/1(ref) -> MATLAB Function/1(ref)
  f32_SpdLimitPos/1 -> Ratelimit/2(f32_SpdLimitPos)
  f32_SpdLimitNeg/1 -> Ratelimit/3(f32_SpdLimitNeg)
  Subsystem1/1(Ki) -> MATLAB Function/4(ki)
  Gain/1 -> "Iqref "/1
  Constant/1 -> Idref/1
  MATLAB Function/2(intgout) -> Unit Delay/1
  Unit Delay/1 -> MATLAB Function/7(intgin)

== system bldc0/bldc/Switch Case Action Subsystem ==
  Input : Inport
  Input1 : Inport  Port=2
  Action Port : ActionPort  ActionPortLabel=case [ IsCtrl ]:
  "Idref " : Outport  VectorParamsAs1DForOutWhenUnconnected=off
  Iqref : Outport  Port=2  VectorParamsAs1DForOutWhenUnconnected=off
  wires:
  Input/1 -> "Idref "/1
  Input1/1 -> Iqref/1

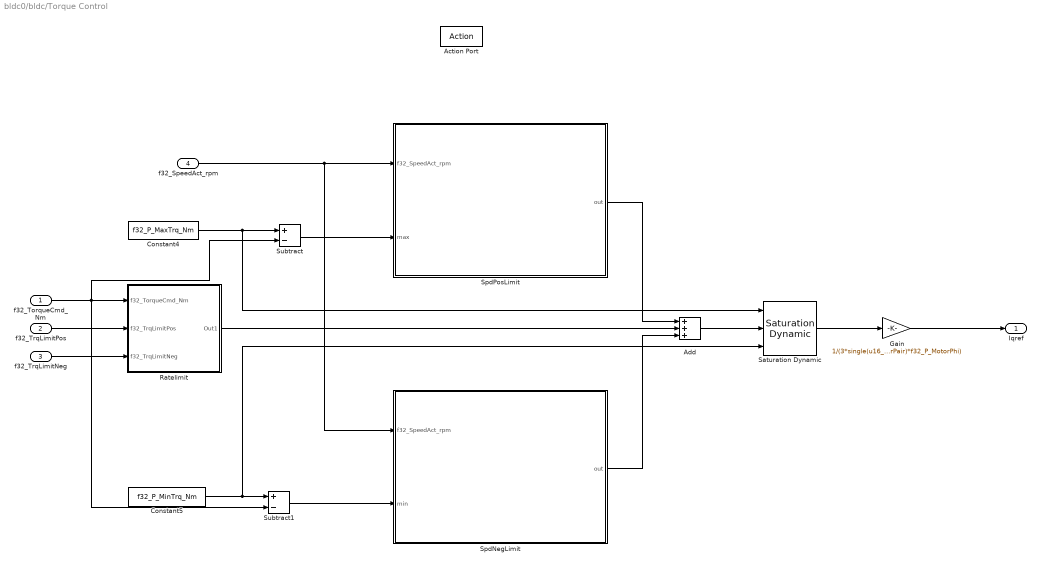
== system bldc0/bldc/Torque Control ==
  f32_TorqueCmd_Nm : Inport
  f32_TrqLimitPos : Inport  Port=2
  f32_TrqLimitNeg : Inport  Port=3
  f32_SpeedAct_rpm : Inport  Port=4
  Action Port : ActionPort  InitializeStates=reset  ActionPortLabel=case [ TrqCtrl ]:
  Add : Sum  Inputs=+++
  Constant4 : Constant  Value=f32_P_MaxTrq_Nm
  Constant5 : Constant  Value=f32_P_MinTrq_Nm
  Gain : Gain  Gain=1/(3*single(u16_P_MotorPair)*f32_P_MotorPhi)  ParamDataTypeStr=single  OutDataTypeStr=single
  Ratelimit : Subsystem
  Saturation Dynamic : simulink/Discontinuities/Saturation Dynamic  OutMin=[]  OutMax=[]  OutDataTypeStr=Inherit: Same as second input  OutDataType=fixdt(1, 16)  OutScaling=2^-10  DoSatur=off
  SpdNegLimit : Subsystem
  SpdPosLimit : Subsystem
  Subtract : Sum  Inputs=+-
  Subtract1 : Sum  Inputs=+-
  Iqref : Outport  InitialOutput=0  VectorParamsAs1DForOutWhenUnconnected=off
  wires:
  Gain/1 -> Iqref/1
  f32_TorqueCmd_Nm/1 -> Subtract1/2, Subtract/2, Ratelimit/1(f32_TorqueCmd_Nm)
  Saturation Dynamic/1 -> Gain/1
  f32_TrqLimitPos/1 -> Ratelimit/2(f32_TrqLimitPos)
  f32_TrqLimitNeg/1 -> Ratelimit/3(f32_TrqLimitNeg)
  f32_SpeedAct_rpm/1 -> SpdNegLimit/1(f32_SpeedAct_rpm), SpdPosLimit/1(f32_SpeedAct_rpm)
  Ratelimit/1(Out1) -> Add/2
  Constant4/1 -> Saturation Dynamic/1, Subtract/1
  Constant5/1 -> Saturation Dynamic/3, Subtract1/1
  Subtract/1 -> SpdPosLimit/2(max)
  Subtract1/1 -> SpdNegLimit/2(min)
  Add/1 -> Saturation Dynamic/2
  SpdPosLimit/1(out) -> Add/1
  SpdNegLimit/1(out) -> Add/3

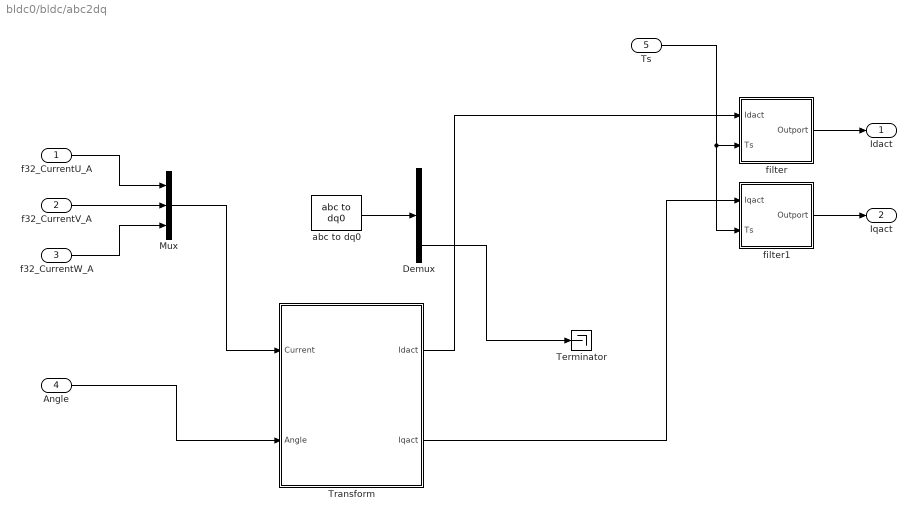
== system bldc0/bldc/abc2dq ==
  f32_CurrentU_A : Inport
  f32_CurrentV_A : Inport  Port=2
  f32_CurrentW_A : Inport  Port=3
  Angle : Inport  Port=4
  Ts : Inport  Port=5
  Demux : Demux  Outputs=3
  Mux : Mux  Inputs=3
  Terminator : Terminator
  Transform : Subsystem
  abc to dq0 : spsabctodq0Lib/abc to dq0  Alignment=Aligned with phase A axis
  filter : Subsystem
  filter1 : Subsystem
  Idact : Outport  VectorParamsAs1DForOutWhenUnconnected=off
  Iqact : Outport  Port=2  VectorParamsAs1DForOutWhenUnconnected=off
  wires:
  Demux/3 -> Terminator/1
  Transform/2(Iqact) -> filter1/1(Iqact)
  Transform/1(Idact) -> filter/1(Idact)
  abc to dq0/1 -> Demux/1
  Mux/1 -> Transform/1(Current)
  f32_CurrentW_A/1 -> Mux/3
  f32_CurrentV_A/1 -> Mux/2
  f32_CurrentU_A/1 -> Mux/1
  Angle/1 -> Transform/2(Angle)
  filter/1(Outport) -> Idact/1
  filter1/1(Outport) -> Iqact/1
  Ts/1 -> filter/2(Ts), filter1/2(Ts)

== system bldc0/bldc/AngleComp/filter1 ==
  In : Inport
  Constant : Constant  OutDataTypeStr=single
  Constant1 : Constant  Value=0.005  OutDataTypeStr=single
  Minus : Sum  Inputs=+-
  Plus : Sum
  Product : Product
  Product1 : Product
  Unit Delay : UnitDelay  SampleTime=-1  HasFrameUpgradeWarning=on
  Outport : Outport
  wires:
  Constant/1 -> Minus/1
  Constant1/1 -> Product/1, Minus/2
  In/1 -> Product/2
  Product/1 -> Plus/2
  Minus/1 -> Product1/2
  Product1/1 -> Plus/1
  Plus/1 -> Unit Delay/1, Outport/1
  Unit Delay/1 -> Product1/1

== system bldc0/bldc/CurrentLoop/Fwd ==
  In1 : Inport
  In2 : Inport  Port=2
  Constant : Constant  Value=u16_P_MotorPair
  Constant1 : Constant  Value=60  OutDataTypeStr=single
  Constant2 : Constant  Value=f32_P_MotorPhi
  Constant3 : Constant  Value=2*pi  OutDataTypeStr=single
  Constant4 : Constant  Value=6  OutDataTypeStr=single
  Divide : Product  Inputs=*/
  Divide1 : Product  Inputs=*/
  Product : Product  OutDataTypeStr=single
  Product1 : Product  Inputs=3
  Product2 : Product
  Sqrt : Sqrt
  Out1 : Outport  VectorParamsAs1DForOutWhenUnconnected=off
  wires:
  Divide1/1 -> Out1/1
  In2/1 -> Divide1/2
  Product2/1 -> Divide1/1
  Product1/1 -> Product2/1
  Sqrt/1 -> Product2/2
  Constant4/1 -> Sqrt/1
  Constant3/1 -> Product1/3
  Constant2/1 -> Product1/2
  Divide/1 -> Product1/1
  Constant1/1 -> Divide/2
  Product/1 -> Divide/1
  In1/1 -> Product/1
  Constant/1 -> Product/2

== system bldc0/bldc/CurrentLoop/Subsystem ==
  In1 : Inport
  Constant : Constant  Value=0.1  OutDataTypeStr=single
  Constant1 : Constant  OutDataTypeStr=single
  Minus : Sum  Inputs=+-
  Plus : Sum
  Product : Product
  Product1 : Product
  Unit Delay : UnitDelay  SampleTime=-1  HasFrameUpgradeWarning=on
  Out1 : Outport
  wires:
  Unit Delay/1 -> Product1/1
  Product1/1 -> Plus/1
  Product/1 -> Plus/2
  Plus/1 -> Out1/1, Unit Delay/1
  Minus/1 -> Product1/2
  Constant1/1 -> Minus/1
  Constant/1 -> Minus/2, Product/1
  In1/1 -> Product/2

== system bldc0/bldc/FWC/PI ==
  Ref : Inport
  Fbk : Inport  Port=2
  Constant : Constant  Value=f32_P_fwcKp/4
  Constant1 : Constant  Value=f32_P_fwcKp
  Constant2 : Constant  Value=f32_P_fwcKi/4
  Constant3 : Constant  Value=f32_P_fwcKi
  Subtract : Sum  Inputs=+-  OutDataTypeStr=single
  Switch : Switch  Criteria=u2 > Threshold  SaturateOnIntegerOverflow=off  InputSameDT=off
  Switch1 : Switch  Criteria=u2 > Threshold  SaturateOnIntegerOverflow=off  InputSameDT=off
  Kp : Outport  VectorParamsAs1DForOutWhenUnconnected=off
  Ki : Outport  Port=2  VectorParamsAs1DForOutWhenUnconnected=off
  wires:
  Constant3/1 -> Switch1/3
  Constant1/1 -> Switch/3
  Constant2/1 -> Switch1/1
  Constant/1 -> Switch/1
  Subtract/1 -> Switch/2, Switch1/2
  Switch1/1 -> Ki/1
  Switch/1 -> Kp/1
  Fbk/1 -> Subtract/2
  Ref/1 -> Subtract/1

== system bldc0/bldc/FWC/Subsystem ==
  Ud : Inport
  Uq : Inport  Port=2
  Add : Sum
  Product : Product
  Product1 : Product
  Sqrt : Sqrt
  Act : Outport  VectorParamsAs1DForOutWhenUnconnected=off
  wires:
  Uq/1 -> Product1/1, Product1/2
  Product/1 -> Add/1
  Ud/1 -> Product/1, Product/2
  Product1/1 -> Add/2
  Sqrt/1 -> Act/1
  Add/1 -> Sqrt/1

== system bldc0/bldc/FWC/filter ==
  In : Inport
  Ts : Inport  Port=2
  Constant : Constant  OutDataTypeStr=single
  Constant1 : Constant  Value=500  OutDataTypeStr=single
  Minus : Sum  Inputs=+-
  Plus : Sum
  Product : Product
  Product1 : Product
  Product2 : Product
  Unit Delay : UnitDelay  SampleTime=-1  HasFrameUpgradeWarning=on
  Outport : Outport
  wires:
  Constant/1 -> Minus/1
  Product2/1 -> Minus/2, Product/1
  In/1 -> Product/2
  Product/1 -> Plus/2
  Minus/1 -> Product1/2
  Product1/1 -> Plus/1
  Plus/1 -> Unit Delay/1, Outport/1
  Unit Delay/1 -> Product1/1
  Constant1/1 -> Product2/1
  Ts/1 -> Product2/2

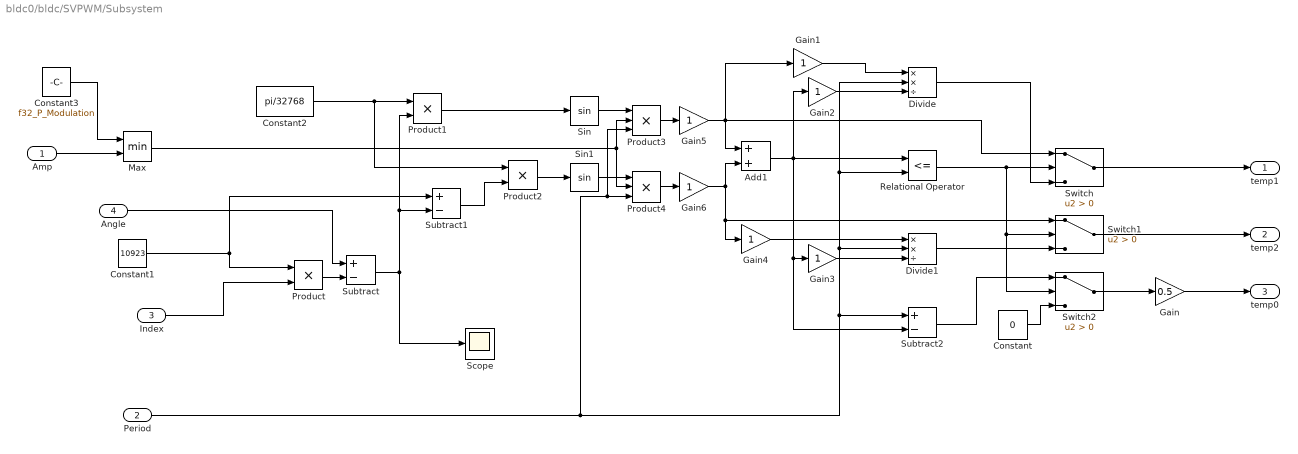
== system bldc0/bldc/SVPWM/Subsystem ==
  Amp : Inport
  Period : Inport  Port=2
  Index : Inport  Port=3
  Angle : Inport  Port=4
  Add1 : Sum
  Constant : Constant  Value=0  OutDataTypeStr=int32
  Constant1 : Constant  Value=10923  OutDataTypeStr=uint32
  Constant2 : Constant  Value=pi/32768  OutDataTypeStr=single
  Constant3 : Constant  Value=f32_P_Modulation  OutDataTypeStr=single
  Divide : Product  Inputs=**/  OutDataTypeStr=int32
  Divide1 : Product  Inputs=**/  OutDataTypeStr=int32
  Gain : Gain  Gain=0.5  OutDataTypeStr=int32
  Gain{1..4} (4 alike) : Gain  OutDataTypeStr=uint32
  Gain5 : Gain  OutDataTypeStr=int32
  Gain6 : Gain  OutDataTypeStr=int32
  Max : MinMax  Inputs=2  OutDataTypeStr=single
  Product : Product
  Product1 : Product  OutDataTypeStr=single
  Product2 : Product  OutDataTypeStr=single
  Product3 : Product  Inputs=3  OutDataTypeStr=single
  Product4 : Product  Inputs=3  OutDataTypeStr=single
  Relational Operator : RelationalOperator  Operator=<=  OutDataTypeStr=boolean  RndMeth=Simplest  InputSameDT=off
  Scope : Scope
  Sin : Trigonometry  OutputSignalType=real
  Sin1 : Trigonometry  OutputSignalType=real
  Subtract : Sum  Inputs=+-  AccumDataTypeStr=uint16
  Subtract1 : Sum  Inputs=+-  AccumDataTypeStr=uint16
  Subtract2 : Sum  Inputs=+-  OutDataTypeStr=int32
  Switch : Switch  Criteria=u2 > Threshold  SaturateOnIntegerOverflow=off  InputSameDT=off
  Switch1 : Switch  Criteria=u2 > Threshold  SaturateOnIntegerOverflow=off  InputSameDT=off
  Switch2 : Switch  Criteria=u2 > Threshold  SaturateOnIntegerOverflow=off  InputSameDT=off
  temp1 : Outport  VectorParamsAs1DForOutWhenUnconnected=off
  temp2 : Outport  Port=2  VectorParamsAs1DForOutWhenUnconnected=off
  temp0 : Outport  Port=3  VectorParamsAs1DForOutWhenUnconnected=off
  wires:
  Period/1 -> Relational Operator/2, Divide/2, Divide1/2, Subtract2/1, Product3/3, Product4/3
  Product3/1 -> Gain5/1
  Product/1 -> Subtract/2
  Subtract/1 -> Scope/1, Subtract1/2, Product1/2
  Add1/1 -> Gain2/1, Relational Operator/1, Gain3/1, Subtract2/2
  Constant2/1 -> Product1/1, Product2/1
  Product1/1 -> Sin/1
  Switch2/1 -> Gain/1
  Subtract2/1 -> Switch2/1
  Index/1 -> Product/2
  Constant/1 -> Switch2/3
  Relational Operator/1 -> Switch/2, Switch1/2, Switch2/2
  Subtract1/1 -> Product2/2
  Product4/1 -> Gain6/1
  Switch/1 -> temp1/1
  Product2/1 -> Sin1/1
  Constant1/1 -> Subtract1/1, Product/1
  Switch1/1 -> temp2/1
  Divide/1 -> Switch/3
  Max/1 -> Product3/2, Product4/2
  Gain/1 -> temp0/1
  Divide1/1 -> Switch1/3
  Amp/1 -> Max/2
  Constant3/1 -> Max/1
  Sin/1 -> Product3/1
  Sin1/1 -> Product4/1
  Gain1/1 -> Divide/1
  Gain2/1 -> Divide/3
  Gain3/1 -> Divide1/3
  Gain4/1 -> Divide1/1
  Gain5/1 -> Add1/1, Switch/1, Gain1/1
  Gain6/1 -> Add1/2, Switch1/1, Gain4/1
  Angle/1 -> Subtract/1

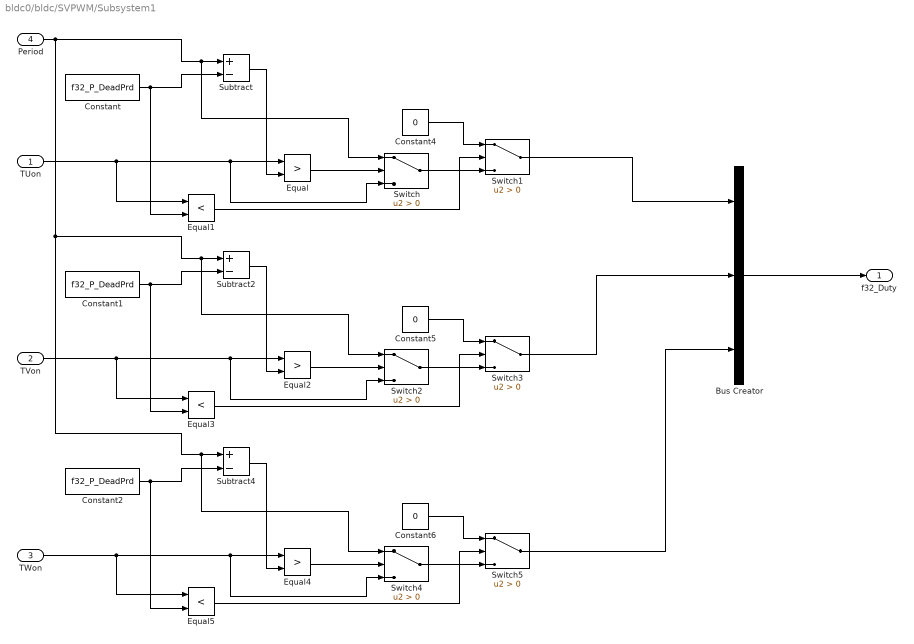
== system bldc0/bldc/SVPWM/Subsystem1 ==
  TUon : Inport
  TVon : Inport  Port=2
  TWon : Inport  Port=3
  Period : Inport  Port=4
  Bus Creator : BusCreator  Inputs=3  OutDataTypeStr=Bus: Duty  NonVirtualBus=on
      settings: InheritFromInputs=off
  Constant : Constant  Value=f32_P_DeadPrd
  Constant1 : Constant  Value=f32_P_DeadPrd
  Constant2 : Constant  Value=f32_P_DeadPrd
  Constant4 : Constant  Value=0  OutDataTypeStr=single
  Constant5 : Constant  Value=0  OutDataTypeStr=single
  Constant6 : Constant  Value=0  OutDataTypeStr=single
  Equal : RelationalOperator  Operator=>  OutDataTypeStr=boolean  RndMeth=Simplest  InputSameDT=off
  Equal1 : RelationalOperator  Operator=<  OutDataTypeStr=boolean  RndMeth=Simplest  InputSameDT=off
  Equal2 : RelationalOperator  Operator=>  OutDataTypeStr=boolean  RndMeth=Simplest  InputSameDT=off
  Equal3 : RelationalOperator  Operator=<  OutDataTypeStr=boolean  RndMeth=Simplest  InputSameDT=off
  Equal4 : RelationalOperator  Operator=>  OutDataTypeStr=boolean  RndMeth=Simplest  InputSameDT=off
  Equal5 : RelationalOperator  Operator=<  OutDataTypeStr=boolean  RndMeth=Simplest  InputSameDT=off
  Subtract : Sum  Inputs=+-
  Subtract2 : Sum  Inputs=+-
  Subtract4 : Sum  Inputs=+-
  Switch{,2..5} (5 alike) : Switch  Criteria=u2 > Threshold  SaturateOnIntegerOverflow=off  InputSameDT=off
  Switch1 : Switch  Criteria=u2 > Threshold  OutDataTypeStr=single  SaturateOnIntegerOverflow=off  InputSameDT=off
  f32_Duty : Outport  OutDataTypeStr=Bus: Duty
  wires:
  Constant/1 -> Equal1/2, Subtract/2
  Subtract/1 -> Equal/2
  Equal/1 -> Switch/2
  TUon/1 -> Equal1/1, Switch/3, Equal/1
  Equal1/1 -> Switch1/2
  Switch/1 -> Switch1/3
  Subtract2/1 -> Equal2/2
  Equal3/1 -> Switch3/2
  Equal2/1 -> Switch2/2
  TVon/1 -> Equal3/1, Switch2/3, Equal2/1
  Switch2/1 -> Switch3/3
  Constant1/1 -> Equal3/2, Subtract2/2
  Subtract4/1 -> Equal4/2
  Equal5/1 -> Switch5/2
  Equal4/1 -> Switch4/2
  TWon/1 -> Equal5/1, Switch4/3, Equal4/1
  Switch4/1 -> Switch5/3
  Constant2/1 -> Equal5/2, Subtract4/2
  Period/1 -> Switch4/1, Subtract4/1, Switch2/1, Subtract2/1, Switch/1, Subtract/1
  Bus Creator/1 -> f32_Duty/1
  Switch1/1 -> Bus Creator/1
  Constant4/1 -> Switch1/1
  Switch3/1 -> Bus Creator/2
  Constant5/1 -> Switch3/1
  Switch5/1 -> Bus Creator/3
  Constant6/1 -> Switch5/1

== system bldc0/bldc/SVPWM/Subsystem2 ==
  In1 : Inport
  Uq : Inport  Port=2
  Ud : Inport  Port=3
  Add2 : Sum  AccumDataTypeStr=uint16
  Atan2 : Trigonometry  Operator=atan2
  Cast To Single : DataTypeConversion  OutDataTypeStr=uint16  SaturateOnIntegerOverflow=off  RndMeth=Floor
  Gain : Gain  Gain=10430.37835  OutDataTypeStr=single
  Gain1 : Gain  OutDataTypeStr=int16
  Angle : Outport
  wires:
  Atan2/1 -> Gain/1
  Cast To Single/1 -> Add2/1
  Uq/1 -> Atan2/1
  In1/1 -> Add2/2
  Ud/1 -> Atan2/2
  Add2/1 -> Angle/1
  Gain/1 -> Gain1/1
  Gain1/1 -> Cast To Single/1

== system bldc0/bldc/SVPWM/Switch Case Action Subsystem ==
  PeriodValue : Inport
  temp0 : Inport  Port=2
  temp1 : Inport  Port=3
  temp2 : Inport  Port=4
  Action Port : ActionPort  ActionPortLabel=case [ 0 ]:
  Subtract : Sum  Inputs=+-  OutDataTypeStr=uint32
  Subtract1 : Sum  Inputs=+-  OutDataTypeStr=uint32
  Subtract2 : Sum  Inputs=+-  OutDataTypeStr=uint32
  Out1 : Outport  OutDataTypeStr=uint32  VectorParamsAs1DForOutWhenUnconnected=off
  Out2 : Outport  Port=2  OutDataTypeStr=uint32  VectorParamsAs1DForOutWhenUnconnected=off
  Out3 : Outport  Port=3  OutDataTypeStr=uint32  VectorParamsAs1DForOutWhenUnconnected=off
  wires:
  Subtract/1 -> Subtract1/1, Out1/1
  Subtract2/1 -> Out3/1
  temp1/1 -> Subtract2/2
  PeriodValue/1 -> Subtract/1
  Subtract1/1 -> Subtract2/1, Out2/1
  temp0/1 -> Subtract/2
  temp2/1 -> Subtract1/2

== system bldc0/bldc/SVPWM/Switch Case Action Subsystem1 ==
  PeriodValue : Inport
  temp0 : Inport  Port=2
  temp1 : Inport  Port=3
  temp2 : Inport  Port=4
  Action Port : ActionPort  ActionPortLabel=case [ 1 ]:
  Subtract : Sum  Inputs=+-  OutDataTypeStr=uint32
  Subtract1 : Sum  Inputs=+-  OutDataTypeStr=uint32
  Subtract2 : Sum  Inputs=+-  OutDataTypeStr=uint32
  Out1 : Outport  OutDataTypeStr=uint32  VectorParamsAs1DForOutWhenUnconnected=off
  Out2 : Outport  Port=2  OutDataTypeStr=uint32  VectorParamsAs1DForOutWhenUnconnected=off
  Out3 : Outport  Port=3  OutDataTypeStr=uint32  VectorParamsAs1DForOutWhenUnconnected=off
  wires:
  Subtract/1 -> Subtract1/1, Out2/1
  Subtract2/1 -> Out3/1
  PeriodValue/1 -> Subtract/1
  temp0/1 -> Subtract/2
  temp1/1 -> Subtract1/2
  temp2/1 -> Subtract2/2
  Subtract1/1 -> Subtract2/1, Out1/1

== system bldc0/bldc/SVPWM/Switch Case Action Subsystem2 ==
  PeriodValue : Inport
  temp0 : Inport  Port=2
  temp1 : Inport  Port=3
  temp2 : Inport  Port=4
  Action Port : ActionPort  ActionPortLabel=case [ 2 ]:
  Subtract : Sum  Inputs=+-  OutDataTypeStr=uint32
  Subtract1 : Sum  Inputs=+-  OutDataTypeStr=uint32
  Subtract2 : Sum  Inputs=+-  OutDataTypeStr=uint32
  Out1 : Outport  OutDataTypeStr=uint32  VectorParamsAs1DForOutWhenUnconnected=off
  Out2 : Outport  Port=2  OutDataTypeStr=uint32  VectorParamsAs1DForOutWhenUnconnected=off
  Out3 : Outport  Port=3  OutDataTypeStr=uint32  VectorParamsAs1DForOutWhenUnconnected=off
  wires:
  Subtract1/1 -> Subtract2/1, Out3/1
  PeriodValue/1 -> Subtract/1
  temp2/1 -> Subtract1/2
  Subtract/1 -> Subtract1/1, Out2/1
  temp0/1 -> Subtract/2
  temp1/1 -> Subtract2/2
  Subtract2/1 -> Out1/1

== system bldc0/bldc/SVPWM/Switch Case Action Subsystem3 ==
  PeriodValue : Inport
  temp0 : Inport  Port=2
  temp1 : Inport  Port=3
  temp2 : Inport  Port=4
  Action Port : ActionPort  ActionPortLabel=case [ 3 ]:
  Subtract : Sum  Inputs=+-  OutDataTypeStr=uint32
  Subtract1 : Sum  Inputs=+-  OutDataTypeStr=uint32
  Subtract2 : Sum  Inputs=+-  OutDataTypeStr=uint32
  Out1 : Outport  OutDataTypeStr=uint32  VectorParamsAs1DForOutWhenUnconnected=off
  Out2 : Outport  Port=2  OutDataTypeStr=uint32  VectorParamsAs1DForOutWhenUnconnected=off
  Out3 : Outport  Port=3  OutDataTypeStr=uint32  VectorParamsAs1DForOutWhenUnconnected=off
  wires:
  temp1/1 -> Subtract1/2
  PeriodValue/1 -> Subtract/1
  temp2/1 -> Subtract2/2
  Subtract2/1 -> Out1/1
  temp0/1 -> Subtract/2
  Subtract/1 -> Subtract1/1, Out3/1
  Subtract1/1 -> Out2/1, Subtract2/1

== system bldc0/bldc/SVPWM/Switch Case Action Subsystem4 ==
  PeriodValue : Inport
  temp0 : Inport  Port=2
  temp1 : Inport  Port=3
  temp2 : Inport  Port=4
  Action Port : ActionPort  ActionPortLabel=case [ 4 ]:
  Subtract : Sum  Inputs=+-  OutDataTypeStr=uint32
  Subtract1 : Sum  Inputs=+-  OutDataTypeStr=uint32
  Subtract2 : Sum  Inputs=+-  OutDataTypeStr=uint32
  Out1 : Outport  OutDataTypeStr=uint32  VectorParamsAs1DForOutWhenUnconnected=off
  Out2 : Outport  Port=2  OutDataTypeStr=uint32  VectorParamsAs1DForOutWhenUnconnected=off
  Out3 : Outport  Port=3  OutDataTypeStr=uint32  VectorParamsAs1DForOutWhenUnconnected=off
  wires:
  Subtract/1 -> Out3/1, Subtract1/1
  temp2/1 -> Subtract1/2
  PeriodValue/1 -> Subtract/1
  Subtract2/1 -> Out2/1
  temp0/1 -> Subtract/2
  Subtract1/1 -> Subtract2/1, Out1/1
  temp1/1 -> Subtract2/2

== system bldc0/bldc/SVPWM/Switch Case Action Subsystem5 ==
  PeriodValue : Inport
  temp0 : Inport  Port=2
  temp1 : Inport  Port=3
  temp2 : Inport  Port=4
  Action Port : ActionPort  ActionPortLabel=case [ 5 ]:
  Subtract : Sum  Inputs=+-  OutDataTypeStr=uint32
  Subtract1 : Sum  Inputs=+-  OutDataTypeStr=uint32
  Subtract2 : Sum  Inputs=+-  OutDataTypeStr=uint32
  Out1 : Outport  OutDataTypeStr=uint32  VectorParamsAs1DForOutWhenUnconnected=off
  Out2 : Outport  Port=2  OutDataTypeStr=uint32  VectorParamsAs1DForOutWhenUnconnected=off
  Out3 : Outport  Port=3  OutDataTypeStr=uint32  VectorParamsAs1DForOutWhenUnconnected=off
  wires:
  Subtract/1 -> Subtract1/1, Out1/1
  temp0/1 -> Subtract/2
  PeriodValue/1 -> Subtract/1
  Subtract1/1 -> Subtract2/1, Out3/1
  Subtract2/1 -> Out2/1
  temp1/1 -> Subtract1/2
  temp2/1 -> Subtract2/2
